simulink library "UAVdesign_net"  (Simulink 7.7)
settings: Solver=ode45  SolverMode=SingleTasking  StartTime=0.0  StopTime=10.0  RelTol=1e-3
undefined symbols (not defined in the file or in its folder): alpha_IERA_IELA_IELA, R_IERA_RA_RA
libraries: UAVdesign_net x75, simulink x13
(part 3 of 8)

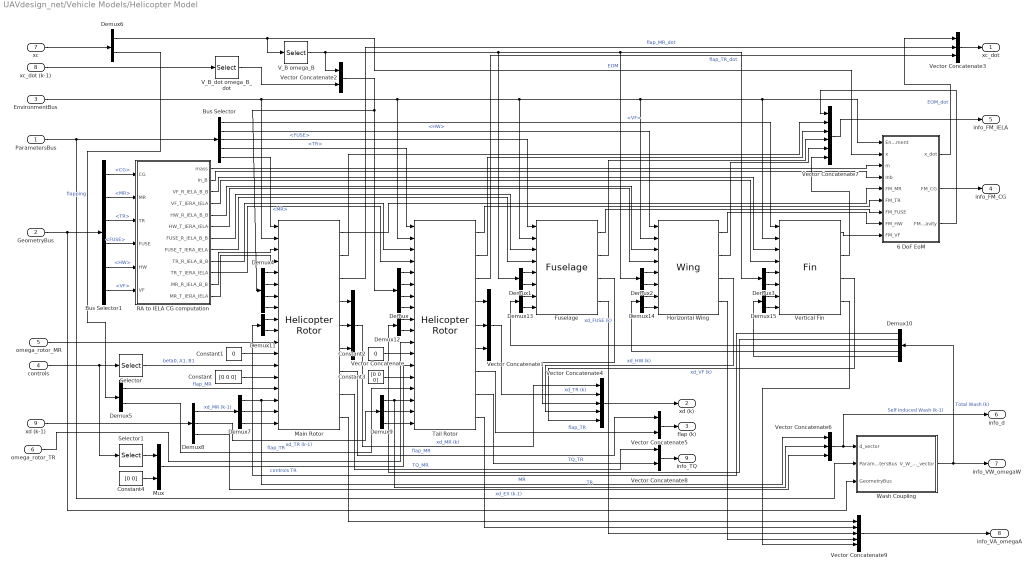
== system UAVdesign_net/Vehicle Models/Helicopter Model ==
  ParametersBus : Inport
  GeometryBus : Inport  Port=2
  EnvironmentBus : Inport  Port=3  OutDataTypeStr=Bus: Environment
  controls : Inport  Port=4
  omega_rotor_MR : Inport  Port=5
  omega_rotor_TR : Inport  Port=6
  xc : Inport  Port=7
  xc_dot (k-1) : Inport  Port=8
  xd (k-1) : Inport  Port=9
  6 DoF EoM : Subsystem
  Bus Selector : BusSelector  OutputSignals=VF,HW,FUSE,TR,MR
  Bus Selector1 : BusSelector  OutputSignals=CG,MR,TR,FUSE,HW,VF
  Constant : Constant  Value=[0 0 0]
  Constant1 : Constant  Value=0
  Constant2 : Constant  Value=0
  Constant3 : Constant  Value=[0 0 0]
  Constant4 : Constant  Value=[0 0]
  Demux : Demux
  Demux{1..3,5,11..15} (9 alike) : Demux  Outputs=2
  Demux10 : Demux  Outputs=[6 6 6 6 6]
  Demux4 : Demux
  Demux6 : Demux  Outputs=[20 6]
  Demux7 : Demux  Outputs=[3 1 1]
  Demux8 : Demux  Outputs=[5 5 9]
  Demux9 : Demux  Outputs=[3 1 1]
  Fuselage : UAVdesign_net/Subsystem Models/Fuselage  SystemSampleTime=-1
  Horizontal Wing : UAVdesign_net/Subsystem Models/Wing  SystemSampleTime=-1
  Main Rotor : UAVdesign_net/Subsystem Models/Helicopter Rotor  SystemSampleTime=-1
  Mux : Mux  Inputs=2
  RA to IELA CG computation : Subsystem
      mask Display:
      | port_label('input', 1, 'CG', 'texmode', 'on')
      | port_label('input', 2, 'MR', 'texmode', 'on')
      | port_label('input', 3, 'TR', 'texmode', 'on')
      | port_label('input', 4, 'FUSE', 'texmode', 'on')
      | port_label('input', 5, 'HW', 'texmode', 'on')
      | port_label('input', 6, 'VF', 'texmode', 'on')
      | 
      | port_label('output', 1, 'mass', 'texmode', 'on')
      | port_label('output', 2, 'In_B', 'texmode', 'on')
      | port_label('output', 3, 'VF R_{IELA-B|B}', 'texmode', 'on')
      | port_label('output', 4, 'VF T_{IERA-IELA}', 'texmode', 'on')
      | port_label('output', 5, 'HW R_{IELA-B|B}', 'texmode', 'on')
      | port_label('output', 6, 'HW T_{IERA-IELA}', 'texmode', 'on')
      | port_label('output', 7, 'FUSE R_{IELA-B|B}', 'texmode', 'on')
      | port_label('output', 8, 'FUSE T_{IERA-IELA}', 'texmode', 'on')
      | port_label('output', 9, 'TR R_{IELA-B|B}', 'texmode', 'on')
      | port_label('output', 10, 'TR T_{IERA-IELA}', 'texmode', 'on')
      | port_label('output', 11, 'MR R_{IELA-B|B}', 'texmode', 'on')
      | port_label('output', 12, 'MR T_{IERA-IELA}', 'texmode', 'on')
  Selector : Selector  InputPortWidth=4  IndexOptions=Index vector (dialog)  Indices=[1:3]  OutputSizes=1
  Selector1 : Selector  InputPortWidth=4  IndexOptions=Index vector (dialog)  Indices=[4]  OutputSizes=1
  Tail Rotor : UAVdesign_net/Subsystem Models/Helicopter Rotor  SystemSampleTime=-1
  V_B omega_B : Selector  InputPortWidth=20  IndexOptions=Index vector (dialog)  Indices=[9:11 15:17]  OutputSizes=1
  V_B_dot omega_B_dot : Selector  InputPortWidth=26  IndexOptions=Index vector (dialog)  Indices=[9:11 15:17]  OutputSizes=1
  Vector Concatenate{,1,3,6} (4 alike) : Concatenate  NumInputs=3  Mode=Vector
  Vector Concatenate2 : Concatenate  Mode=Vector
  Vector Concatenate4 : Concatenate  NumInputs=5  Mode=Vector
  Vector Concatenate5 : Concatenate  Mode=Vector
  Vector Concatenate7 : Concatenate  NumInputs=6  Mode=Vector
  Vector Concatenate8 : Concatenate  Mode=Vector
  Vector Concatenate9 : Concatenate  NumInputs=5  Mode=Vector
  Vertical Fin : UAVdesign_net/Subsystem Models/Fin  SystemSampleTime=-1
  Wash Coupling : Subsystem
      mask Display:
      | port_label('input', 1, 'd VECT', 'texmode', 'on')
      | port_label('input', 2, 'Param.Bus', 'texmode', 'on')
      | port_label('input', 3, 'Geom.Bus', 'texmode', 'on')
      | 
      | port_label('output', 1, 'V_{W} \omega_{W} VECT', 'texmode', 'on')
  xc_dot : Outport
  xd (k) : Outport  Port=2
  flap (k) : Outport  Port=3
  info_FM_CG : Outport  Port=4
  info_FM_IELA : Outport  Port=5
  info_d : Outport  Port=6
  info_VW_omegaW : Outport  Port=7
  info_VA_omegaA : Outport  Port=8
  info_TQ : Outport  Port=9
  wires:
  Vector Concatenate7/1 -> info_FM_IELA/1
  Vertical Fin/2 -> Vector Concatenate7/6
  Horizontal Wing/2 -> Vector Concatenate7/5
  Fuselage/2 -> Vector Concatenate7/4
  Tail Rotor/2 -> Vector Concatenate7/3
  Main Rotor/2 -> Vector Concatenate7/2
  6 DoF EoM/3(FM_Gravity) -> Vector Concatenate7/1
  Fuselage/3 -> Vector Concatenate4/3  "xd_FUSE (k)"
  Tail Rotor/3 -> Vector Concatenate3/3  "flap_TR_dot"
  Tail Rotor/6 -> Vector Concatenate1/3
  Tail Rotor/5 -> Vector Concatenate1/2
  Tail Rotor/4 -> Vector Concatenate1/1
  Tail Rotor/7 -> Vector Concatenate5/2  "flap_TR"
  Main Rotor/3 -> Vector Concatenate3/2  "flap_MR_dot"
  Main Rotor/6 -> Vector Concatenate/3
  Main Rotor/5 -> Vector Concatenate/2
  Main Rotor/4 -> Vector Concatenate/1
  Main Rotor/7 -> Vector Concatenate5/1  "flap_MR"
  Horizontal Wing/3 -> Vector Concatenate4/4  "xd_HW (k)"
  Vertical Fin/3 -> Vector Concatenate4/5  "xd_VF (k)"
  Demux10/1 -> Demux11/1
  Demux10/2 -> Demux12/1
  Demux10/3 -> Demux13/1
  Demux10/4 -> Demux14/1
  Demux10/5 -> Demux15/1
  Vector Concatenate6/1 -> info_d/1, Wash Coupling/1(d_vector)  "Self Induced Wash (k-1)"
  Wash Coupling/1(V_W_omega_W_vector) -> Demux10/1, info_VW_omegaW/1  "Total Wash (k)"
  Demux15/2 -> Vertical Fin/8
  Demux15/1 -> Vertical Fin/7
  Demux14/2 -> Horizontal Wing/8
  Demux14/1 -> Horizontal Wing/7
  Demux13/2 -> Fuselage/8
  Demux13/1 -> Fuselage/7
  Demux12/2 -> Tail Rotor/10
  Demux12/1 -> Tail Rotor/9
  Demux11/2 -> Main Rotor/10
  Demux11/1 -> Main Rotor/9
  6 DoF EoM/2(FM_CG) -> info_FM_CG/1
  Vector Concatenate5/1 -> flap (k)/1
  Demux1/1 -> Fuselage/5
  Demux1/2 -> Fuselage/6
  Demux3/2 -> Vertical Fin/6
  Demux3/1 -> Vertical Fin/5
  Demux2/2 -> Horizontal Wing/6
  Demux2/1 -> Horizontal Wing/5
  Demux8/3 -> Vector Concatenate6/3  "xd_EX (k-1)"
  xd (k-1)/1 -> Demux8/1
  Vector Concatenate/1 -> Vector Concatenate4/1  "xd_MR (k)"
  Demux8/2 -> Demux9/1  "xd_TR (k-1)"
  Demux8/1 -> Demux7/1  "xd_MR (k-1)"
  Demux5/1 -> Main Rotor/15  "flap_MR"
  Demux9/3 -> Tail Rotor/18
  Demux9/2 -> Tail Rotor/17
  Vector Concatenate4/1 -> xd (k)/1
  Vector Concatenate1/1 -> Vector Concatenate4/2  "xd_TR (k)"
  Demux7/3 -> Main Rotor/18
  Demux7/2 -> Main Rotor/17
  Demux5/2 -> Tail Rotor/15  "flap_TR"
  6 DoF EoM/1(x_dot) -> Vector Concatenate3/1  "EOM_dot"
  Vector Concatenate3/1 -> xc_dot/1
  Vector Concatenate2/1 -> Demux4/1, Demux/1
  V_B_dot omega_B_dot/1 -> Vector Concatenate2/2
  V_B omega_B/1 -> Demux2/1, Demux3/1, Demux1/1, Vector Concatenate2/1
  Demux6/1 -> V_B omega_B/1, 6 DoF EoM/2(x)  "EOM"
  Demux6/2 -> Demux5/1  "flapping"
  xc/1 -> Demux6/1
  xc_dot (k-1)/1 -> V_B_dot omega_B_dot/1
  GeometryBus/1 -> Wash Coupling/3(GeometryBus), Bus Selector1/1
  Bus Selector1/6 -> RA to IELA CG computation/6(VF)  "<VF>"
  Bus Selector1/5 -> RA to IELA CG computation/5(HW)  "<HW>"
  Bus Selector1/4 -> RA to IELA CG computation/4(FUSE)  "<FUSE>"
  Bus Selector1/3 -> RA to IELA CG computation/3(TR)  "<TR>"
  Bus Selector1/2 -> RA to IELA CG computation/2(MR)  "<MR>"
  Bus Selector1/1 -> RA to IELA CG computation/1(CG)  "<CG>"
  EnvironmentBus/1 -> Main Rotor/2, Tail Rotor/2, Fuselage/2, Horizontal Wing/2, Vertical Fin/2, 6 DoF EoM/1(Environment)
  ParametersBus/1 -> Wash Coupling/2(ParametersBus), Bus Selector/1
  Bus Selector/1 -> Vertical Fin/1  "<VF>"
  Bus Selector/2 -> Horizontal Wing/1  "<HW>"
  Bus Selector/3 -> Fuselage/1  "<FUSE>"
  Bus Selector/4 -> Tail Rotor/1  "<TR>"
  Bus Selector/5 -> Main Rotor/1  "<MR>"
  Constant4/1 -> Mux/2
  Selector1/1 -> Mux/1
  Mux/1 -> Tail Rotor/13  "controls TR"
  omega_rotor_TR/1 -> Tail Rotor/11
  Constant3/1 -> Tail Rotor/14
  Constant2/1 -> Tail Rotor/12
  controls/1 -> Selector/1, Selector1/1
  Selector/1 -> Main Rotor/13  "beta0, A1, B1"
  omega_rotor_MR/1 -> Main Rotor/11
  Constant1/1 -> Main Rotor/12
  Constant/1 -> Main Rotor/14
  Demux4/4 -> Main Rotor/8
  Demux4/3 -> Main Rotor/7
  Demux4/2 -> Main Rotor/6
  Demux4/1 -> Main Rotor/5
  Demux/4 -> Tail Rotor/8
  Demux/3 -> Tail Rotor/7
  Demux/2 -> Tail Rotor/6
  Demux/1 -> Tail Rotor/5
  RA to IELA CG computation/10(TR_T_IERA_IELA) -> Tail Rotor/4
  RA to IELA CG computation/9(TR_R_IELA_B_B) -> Tail Rotor/3
  RA to IELA CG computation/8(FUSE_T_IERA_IELA) -> Fuselage/4
  RA to IELA CG computation/7(FUSE_R_IELA_B_B) -> Fuselage/3
  RA to IELA CG computation/6(HW_T_IERA_IELA) -> Horizontal Wing/4
  RA to IELA CG computation/5(HW_R_IELA_B_B) -> Horizontal Wing/3
  RA to IELA CG computation/4(VF_T_IERA_IELA) -> Vertical Fin/4
  RA to IELA CG computation/3(VF_R_IELA_B_B) -> Vertical Fin/3
  Tail Rotor/1 -> 6 DoF EoM/6(FM_TR)
  Fuselage/1 -> 6 DoF EoM/7(FM_FUSE)
  Horizontal Wing/1 -> 6 DoF EoM/8(FM_HW)
  Vertical Fin/1 -> 6 DoF EoM/9(FM_VF)
  Demux9/1 -> Vector Concatenate6/2, Tail Rotor/16  "TR"
  Demux7/1 -> Vector Concatenate6/1, Main Rotor/16  "MR"
  RA to IELA CG computation/2(In_B) -> 6 DoF EoM/4(Inb)
  RA to IELA CG computation/1(mass) -> 6 DoF EoM/3(m)
  Main Rotor/1 -> 6 DoF EoM/5(FM_MR)
  RA to IELA CG computation/11(MR_R_IELA_B_B) -> Main Rotor/3
  RA to IELA CG computation/12(MR_T_IERA_IELA) -> Main Rotor/4
  Tail Rotor/8 -> Vector Concatenate8/2  "TQ_TR"
  Main Rotor/8 -> Vector Concatenate8/1  "TQ_MR"
  Vector Concatenate8/1 -> info_TQ/1
  Main Rotor/9 -> Vector Concatenate9/1
  Tail Rotor/9 -> Vector Concatenate9/2
  Fuselage/4 -> Vector Concatenate9/3
  Horizontal Wing/4 -> Vector Concatenate9/4
  Vertical Fin/4 -> Vector Concatenate9/5
  Vector Concatenate9/1 -> info_VA_omegaA/1

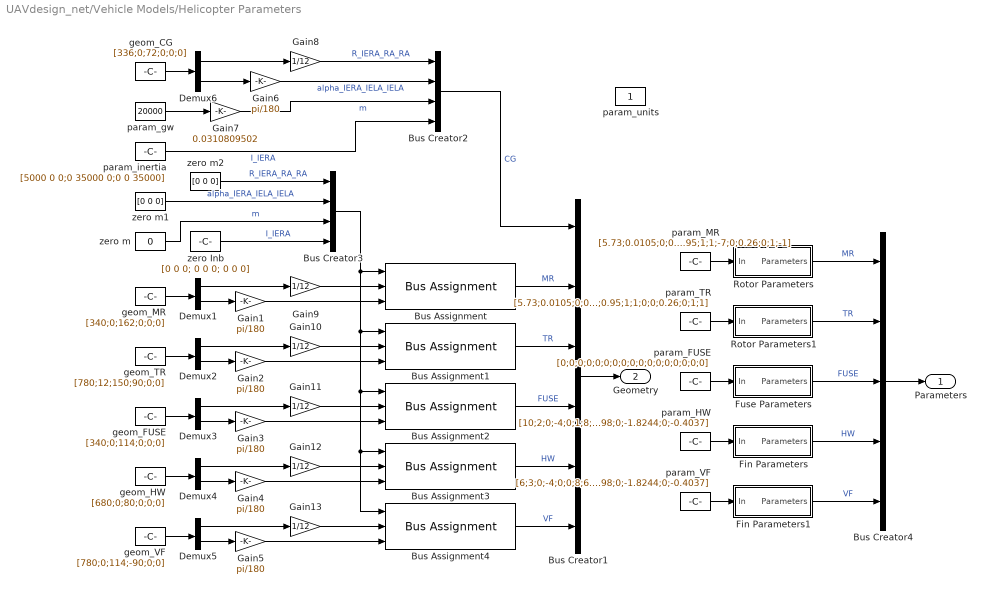
== system UAVdesign_net/Vehicle Models/Helicopter Parameters ==
  Bus Assignment{,1..4} (5 alike) : BusAssignment  AssignedSignals=R_IERA_RA_RA,alpha_IERA_IELA_IELA
  Bus Creator1 : BusCreator  Inputs=6
  Bus Creator2 : BusCreator  OutDataTypeStr=Bus: GeometryParameters
  Bus Creator3 : BusCreator  OutDataTypeStr=Bus: GeometryParameters
  Bus Creator4 : BusCreator  Inputs=5
  Demux{1..6} (6 alike) : Demux  Outputs=2
  Fin Parameters : Subsystem
  Fin Parameters1 : Subsystem
  Fuse Parameters : Subsystem
  Gain{1..6} (6 alike) : Gain  Gain=pi/180
  Gain{8..13} (6 alike) : Gain  Gain=1/12
  Gain7 : Gain  Gain=0.0310809502
  Rotor Parameters : Subsystem
  Rotor Parameters1 : Subsystem
  geom_CG : Constant  Value=[336;0;72;0;0;0]
  geom_FUSE : Constant  Value=[340;0;114;0;0;0]
  geom_HW : Constant  Value=[680;0;80;0;0;0]
  geom_MR : Constant  Value=[340;0;162;0;0;0]
  geom_TR : Constant  Value=[780;12;150;90;0;0]
  geom_VF : Constant  Value=[780;0;114;-90;0;0]
  param_FUSE : Constant  Value=[0;0;0;0;0;0;0;0;0;0;0;0;0;0;0;0;0]
  param_HW : Constant  Value=[10;2;0;-4;0;1;8;6.13;0.9682;1.8898;0;-1.8244;0;-0.4037]
  param_MR : Constant  Value=[5.73;0.0105;0;0.01325;0;-15;0;0;7;30;2.5;0.95;1;1;-7;0;0.26;0;1;-1]
  param_TR : Constant  Value=[5.73;0.0105;0;0.01325;0;-45;0;0;4;6.5;1.25;0.95;1;1;0;0;0.26;0;1;1]
  param_VF : Constant  Value=[6;3;0;-4;0;0;8;6.1311;0.9682;1.8898;0;-1.8244;0;-0.4037]
  param_gw : Constant  Value=20000
  param_inertia : Constant  Value=[5000 0 0;0 35000 0;0 0 35000]
  param_units : Constant
  zero Inb : Constant  Value=[0 0 0; 0 0 0; 0 0 0]
  zero m : Constant  Value=0
  zero m1 : Constant  Value=[0 0 0]
  zero m2 : Constant  Value=[0 0 0]
  Parameters : Outport
  Geometry : Outport  Port=2
  wires:
  Bus Creator2/1 -> Bus Creator1/1  "CG"
  Bus Assignment1/1 -> Bus Creator1/3  "TR"
  Bus Assignment2/1 -> Bus Creator1/4  "FUSE"
  Bus Assignment3/1 -> Bus Creator1/5  "HW"
  Bus Assignment4/1 -> Bus Creator1/6  "VF"
  Bus Creator1/1 -> Geometry/1
  Demux6/1 -> Gain8/1
  Demux6/2 -> Gain6/1
  param_gw/1 -> Gain7/1
  param_inertia/1 -> Bus Creator2/4  "I_IERA"
  Bus Assignment/1 -> Bus Creator1/2  "MR"
  Demux1/1 -> Gain9/1
  Demux1/2 -> Gain1/1
  geom_MR/1 -> Demux1/1
  Demux2/1 -> Gain10/1
  Demux2/2 -> Gain2/1
  geom_TR/1 -> Demux2/1
  Demux3/1 -> Gain11/1
  Demux3/2 -> Gain3/1
  geom_FUSE/1 -> Demux3/1
  Demux4/1 -> Gain12/1
  Demux4/2 -> Gain4/1
  geom_HW/1 -> Demux4/1
  Demux5/1 -> Gain13/1
  Demux5/2 -> Gain5/1
  geom_VF/1 -> Demux5/1
  geom_CG/1 -> Demux6/1
  Bus Creator3/1 -> Bus Assignment/1, Bus Assignment1/1, Bus Assignment2/1, Bus Assignment4/1, Bus Assignment3/1
  zero m/1 -> Bus Creator3/3  "m"
  zero m1/1 -> Bus Creator3/2  "alpha_IERA_IELA_IELA"
  zero Inb/1 -> Bus Creator3/4  "I_IERA"
  zero m2/1 -> Bus Creator3/1  "R_IERA_RA_RA"
  Bus Creator4/1 -> Parameters/1
  Rotor Parameters/1(Parameters) -> Bus Creator4/1  "MR"
  param_MR/1 -> Rotor Parameters/1(In)
  Rotor Parameters1/1(Parameters) -> Bus Creator4/2  "TR"
  param_TR/1 -> Rotor Parameters1/1(In)
  param_FUSE/1 -> Fuse Parameters/1(In)
  Fuse Parameters/1(Parameters) -> Bus Creator4/3  "FUSE"
  param_VF/1 -> Fin Parameters1/1(In)
  Fin Parameters1/1(Parameters) -> Bus Creator4/5  "VF"
  Fin Parameters/1(Parameters) -> Bus Creator4/4  "HW"
  param_HW/1 -> Fin Parameters/1(In)
  Gain1/1 -> Bus Assignment/3
  Gain2/1 -> Bus Assignment1/3
  Gain3/1 -> Bus Assignment2/3
  Gain4/1 -> Bus Assignment3/3
  Gain5/1 -> Bus Assignment4/3
  Gain6/1 -> Bus Creator2/2  "alpha_IERA_IELA_IELA"
  Gain7/1 -> Bus Creator2/3  "m"
  Gain8/1 -> Bus Creator2/1  "R_IERA_RA_RA"
  Gain9/1 -> Bus Assignment/2
  Gain10/1 -> Bus Assignment1/2
  Gain11/1 -> Bus Assignment2/2
  Gain12/1 -> Bus Assignment3/2
  Gain13/1 -> Bus Assignment4/2

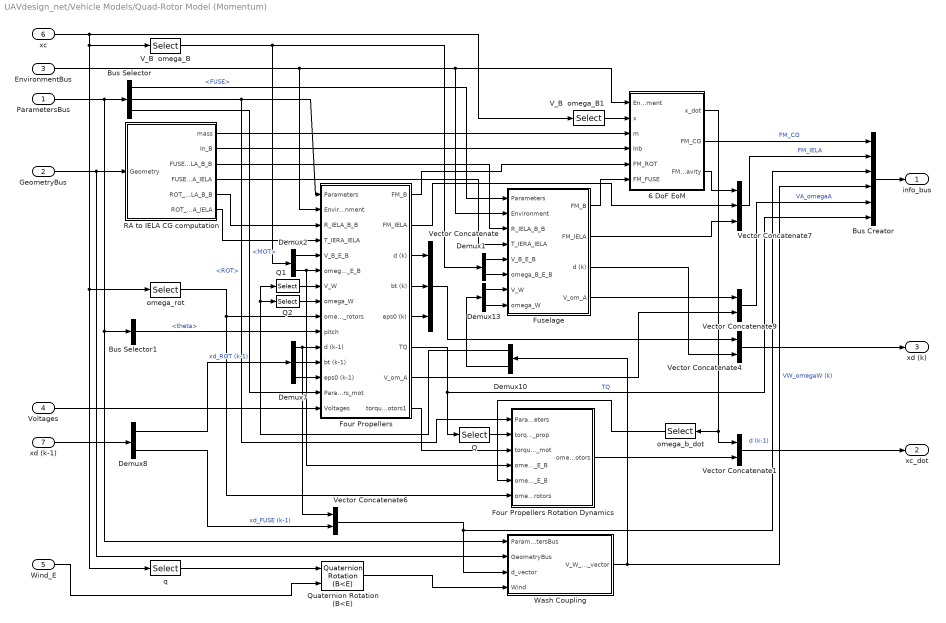
== system UAVdesign_net/Vehicle Models/Quad-Rotor Model (Momentum) ==
  ParametersBus : Inport
  GeometryBus : Inport  Port=2
  EnvironmentBus : Inport  Port=3
  Voltages : Inport  Port=4
  Wind_E : Inport  Port=5
  xc : Inport  Port=6
  xd (k-1) : Inport  Port=7
  6 DoF EoM : Subsystem
  Bus Creator : BusCreator  Inputs=6
  Bus Selector : BusSelector  OutputSignals=FUSE,ROT,MOT
  Bus Selector1 : BusSelector  OutputSignals=ROT.theta
  Demux1 : Demux  Outputs=2
  Demux10 : Demux  Outputs=[24 6]
  Demux13 : Demux  Outputs=2
  Demux2 : Demux  Outputs=2
  Demux7 : Demux  Outputs=[12 4 4]
  Demux8 : Demux  Outputs=[20 3]
  Four Propellers : Subsystem  TreatAsAtomicUnit=on
      mask Display:
      | port_label('input', 1, 'Parameters', 'texmode', 'on')
      | port_label('input', 2, 'Environment', 'texmode', 'on')
      | port_label('input', 3, 'R_{IELA-B|B}', 'texmode', 'on')
      | port_label('input', 4, 'T_{IERA-IELA}', 'texmode', 'on')
      | port_label('input', 5, 'V_{B-E|B}', 'texmode', 'on')
      | port_label('input', 6, '\omega_{B-E|B}', 'texmode', 'on')
      | port_label('input', 7, 'V_{W|B}', 'texmode', 'on')
      | port_label('input', 8, '\omega_{W|B}', 'texmode', 'on')
      | port_label('input', 9, '\Omega_{rotor}', 'texmode', 'on')
      | port_label('input', 10, 'pitch', 'texmode', 'on')
      | port_label('input', 11, 'd_{k-1|IELA}', 'texmode', 'on')
      | port_label('input', 12, 'bt_{k-1}', 'texmode', 'on')
      | port_label('input', 13, 'eps0_{k-1}', 'texmode', 'on')
      | port_label('input', 14, 'Parameters_{mot}', 'texmode', 'on')
      | port_label('input', 15, 'V_{mot}', 'texmode', 'on')
      | 
      | port_label('output', 1, 'FM_{B}', 'texmode', 'on')
      | port_label('output', 2, 'FM_{IELA}', 'texmode', 'on')
      | port_label('output', 3, 'd_{k|IELA}', 'texmode', 'on')
      | port_label('output', 4, 'bt_{k}', 'texmode', 'on')
      | port_label('output', 5, 'eps0_{k}', 'texmode', 'on')
      | port_label('output', 6, 'T Q', 'texmode', 'on')
      | port_label('output', 7, 'V \omega_{A|IELA}', 'texmode', 'on')
      | port_label('output', 8, '\tau_{motor}', 'texmode', 'on')
  Four Propellers Rotation Dynamics : Subsystem  TreatAsAtomicUnit=on
      mask Display:
      | port_label('input', 1, 'Parameters', 'texmode', 'on')
      | port_label('input', 2, '\tau_{prop} (Q)', 'texmode', 'on')
      | port_label('input', 3, '\tau_{motor}', 'texmode', 'on')
      | port_label('input', 4, '\omega_{B-E|B}', 'texmode', 'on')
      | port_label('input', 5, '\omega^\bullet_{B-E|B}', 'texmode', 'on')
      | port_label('input', 6, '\Omega_{rotor}', 'texmode', 'on')
      | 
      | port_label('output', 1, '\Omega^\bullet_{rotor}', 'texmode', 'on')
  Fuselage : Subsystem  TreatAsAtomicUnit=on
      mask Type: HelicopterFuselageModel
      mask Description: Fuselage model.
      mask Display:
      | port_label('input', 1, 'Parameters', 'texmode', 'on')
      | port_label('input', 2, 'Environment', 'texmode', 'on')
      | port_label('input', 3, 'R_{IELA-B|B}', 'texmode', 'on')
      | port_label('input', 4, 'T_{IERA-IELA}', 'texmode', 'on')
      | port_label('input', 5, 'V_{B-E|B}', 'texmode', 'on')
      | port_label('input', 6, '\omega_{B-E|B}', 'texmode', 'on')
      | port_label('input', 7, 'V_{W|B}', 'texmode', 'on')
      | port_label('input', 8, '\omega_{W|B}', 'texmode', 'on')
      | 
      | port_label('output', 1, 'FM_{B}', 'texmode', 'on')
      | port_label('output', 2, 'FM_{IELA}', 'texmode', 'on')
      | port_label('output', 3, 'd_{IELA}', 'texmode', 'on')
      | port_label('output', 4, 'V \omega_{A|IELA}', 'texmode', 'on')
  Q : Selector  InputPortWidth=8  IndexOptions=Index vector (dialog)  Indices=[2 4 6 8]  OutputSizes=1
  Q1 : Selector  InputPortWidth=24  IndexOptions=Index vector (dialog)  Indices=[1:3 7:9 13:15 19:21]  OutputSizes=1
  Q2 : Selector  InputPortWidth=24  IndexOptions=Index vector (dialog)  Indices=[4:6 10:12 16:18 22:24]  OutputSizes=1
  Quaternion Rotation (B<E) : UAVdesign_net/Utilities/Math/Quaternion Rotation (B<E)  SystemSampleTime=-1
  RA to IELA CG computation : Subsystem
      mask Display:
      | port_label('input', 1, 'Geom', 'texmode', 'on')
      | 
      | port_label('output', 1, 'mass', 'texmode', 'on')
      | port_label('output', 2, 'In_B', 'texmode', 'on')
      | port_label('output', 3, 'FUSE R_{IELA-B|B}', 'texmode', 'on')
      | port_label('output', 4, 'FUSE T_{IERA-IELA}', 'texmode', 'on')
      | port_label('output', 5, 'ROT R_{IELA-B|B}', 'texmode', 'on')
      | port_label('output', 6, 'ROT T_{IERA-IELA}', 'texmode', 'on')
  V_B  omega_B : Selector  InputPortWidth=17  IndexOptions=Index vector (dialog)  Indices=[1:6]  OutputSizes=1
  V_B  omega_B1 : Selector  InputPortWidth=17  IndexOptions=Index vector (dialog)  Indices=[1:13]  OutputSizes=1
  Vector Concatenate : Concatenate  NumInputs=3  Mode=Vector
  Vector Concatenate{1,4,6,9} (4 alike) : Concatenate  Mode=Vector
  Vector Concatenate7 : Concatenate  NumInputs=3  Mode=Vector
  Wash Coupling : Subsystem
      mask Display:
      | port_label('input', 1, 'Param.Bus', 'texmode', 'on')
      | port_label('input', 2, 'Geom.Bus', 'texmode', 'on')
      | port_label('input', 3, 'd VECT', 'texmode', 'on')
      | port_label('input', 4, 'wind VECT', 'texmode', 'on')
      | 
      | port_label('output', 1, 'V_{W} \omega_{W} VECT', 'texmode', 'on')
  omega_b_dot : Selector  InputPortWidth=13  IndexOptions=Index vector (dialog)  Indices=[4:6]  OutputSizes=1
  omega_rot : Selector  InputPortWidth=17  IndexOptions=Index vector (dialog)  Indices=[14:17]  OutputSizes=1
  q : Selector  InputPortWidth=17  IndexOptions=Index vector (dialog)  Indices=[10:13]  OutputSizes=1
  info_bus : Outport
  xc_dot : Outport  Port=2
  xd (k) : Outport  Port=3
  wires:
  Vector Concatenate9/1 -> Bus Creator/5  "VA_omegaA"
  Four Propellers/1(FM_B) -> 6 DoF EoM/5(FM_ROT)
  RA to IELA CG computation/1(mass) -> 6 DoF EoM/3(m)
  RA to IELA CG computation/2(In_B) -> 6 DoF EoM/4(Inb)
  Fuselage/1(FM_B) -> 6 DoF EoM/6(FM_FUSE)
  RA to IELA CG computation/3(FUSE_R_IELA_B_B) -> Fuselage/3(R_IELA_B_B)
  RA to IELA CG computation/4(FUSE_T_IERA_IELA) -> Fuselage/4(T_IERA_IELA)
  Bus Selector/2 -> Four Propellers/1(Parameters), Four Propellers Rotation Dynamics/1(Parameters)  "<ROT>"
  Bus Selector/1 -> Fuselage/1(Parameters)  "<FUSE>"
  ParametersBus/1 -> Bus Selector/1, Wash Coupling/1(ParametersBus), Bus Selector1/1
  EnvironmentBus/1 -> Fuselage/2(Environment), 6 DoF EoM/1(Environment), Four Propellers/2(Environment)
  GeometryBus/1 -> Wash Coupling/2(GeometryBus), RA to IELA CG computation/1(Geometry)
  V_B  omega_B/1 -> Demux1/1, Demux2/1
  Vector Concatenate4/1 -> xd (k)/1
  Demux8/1 -> Demux7/1  "xd_ROT (k-1)"
  xd (k-1)/1 -> Demux8/1
  Demux1/2 -> Fuselage/6(omega_B_E_B)
  Demux1/1 -> Fuselage/5(V_B_E_B)
  Demux13/1 -> Fuselage/7(V_W)
  Demux13/2 -> Fuselage/8(omega_W)
  Wash Coupling/1(V_W_omega_W_vector) -> Demux10/1, Bus Creator/4  "VW_omegaW (k)"
  Demux10/1 -> Q1/1, Q2/1
  6 DoF EoM/3(FM_Gravity) -> Vector Concatenate7/1
  Four Propellers/2(FM_IELA) -> Vector Concatenate7/2
  Fuselage/2(FM_IELA) -> Vector Concatenate7/3
  Vector Concatenate7/1 -> Bus Creator/2  "FM_IELA"
  Four Propellers/3(d (k)) -> Vector Concatenate/1
  Fuselage/4(V_om_A) -> Vector Concatenate9/1
  Demux10/2 -> Demux13/1
  Vector Concatenate/1 -> Vector Concatenate4/1
  Fuselage/3(d (k)) -> Vector Concatenate4/2
  Demux8/2 -> Vector Concatenate6/2  "xd_FUSE (k-1)"
  Vector Concatenate6/1 -> Wash Coupling/3(d_vector), Bus Creator/3  "d (k-1)"
  xc/1 -> V_B  omega_B/1, omega_rot/1, q/1, V_B  omega_B1/1
  RA to IELA CG computation/5(ROT_R_IELA_B_B) -> Four Propellers/3(R_IELA_B_B)
  Bus Selector1/1 -> Four Propellers/10(pitch)  "<theta>"
  RA to IELA CG computation/6(ROT_T_IERA_IELA) -> Four Propellers/4(T_IERA_IELA)
  Demux2/1 -> Four Propellers/5(V_B_E_B)
  Demux2/2 -> Four Propellers/6(omega_B_E_B), Four Propellers Rotation Dynamics/4(omega_B_E_B)
  Q1/1 -> Four Propellers/7(V_W)
  Q2/1 -> Four Propellers/8(omega_W)
  Demux7/1 -> Four Propellers/11(d (k-1)), Vector Concatenate6/1
  Demux7/2 -> Four Propellers/12(bt (k-1))
  Demux7/3 -> Four Propellers/13(eps0 (k-1))
  Bus Selector/3 -> Four Propellers/14(Parameters_mot)  "<MOT>"
  Voltages/1 -> Four Propellers/15(Voltages)
  Four Propellers/7(V_om_A) -> Vector Concatenate9/2
  Four Propellers/4(bt (k)) -> Vector Concatenate/2
  Four Propellers/5(eps0 (k)) -> Vector Concatenate/3
  Four Propellers/8(torque_motors1) -> Four Propellers Rotation Dynamics/3(torque_mot)
  Q/1 -> Four Propellers Rotation Dynamics/2(torque_prop)
  Four Propellers/6(TQ) -> Q/1, Bus Creator/6  "TQ"
  6 DoF EoM/1(x_dot) -> Vector Concatenate1/1, omega_b_dot/1
  Vector Concatenate1/1 -> xc_dot/1
  Four Propellers Rotation Dynamics/1(omega_dot_motors) -> Vector Concatenate1/2
  omega_b_dot/1 -> Four Propellers Rotation Dynamics/5(omega_dot_B_E_B)
  omega_rot/1 -> Four Propellers/9(omega_rotors), Four Propellers Rotation Dynamics/6(omega_rotors)
  Bus Creator/1 -> info_bus/1
  6 DoF EoM/2(FM_CG) -> Bus Creator/1  "FM_CG"
  V_B  omega_B1/1 -> 6 DoF EoM/2(x)
  Quaternion Rotation (B<E)/1 -> Wash Coupling/4(Wind)
  Wind_E/1 -> Quaternion Rotation (B<E)/2
  q/1 -> Quaternion Rotation (B<E)/1

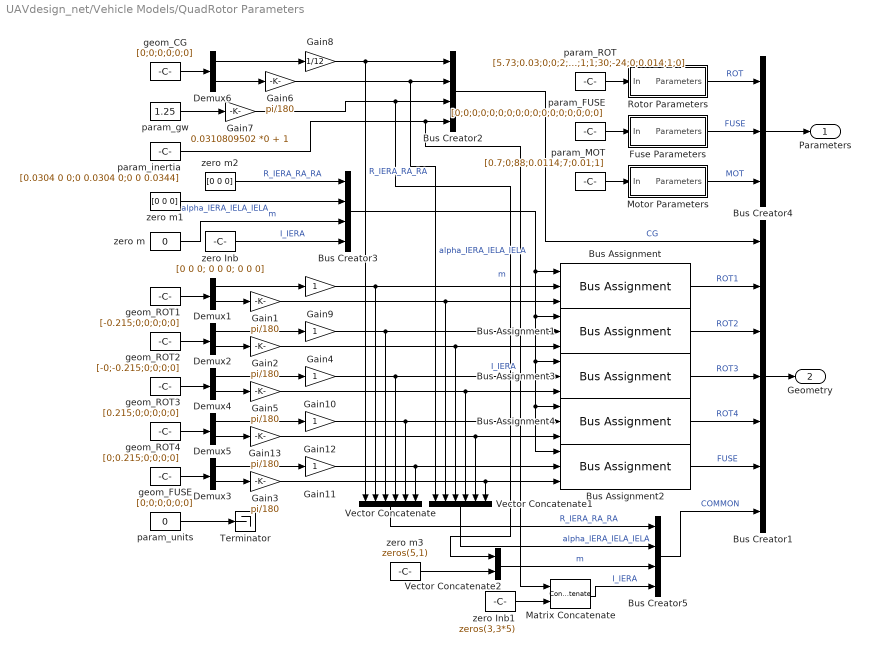
== system UAVdesign_net/Vehicle Models/QuadRotor Parameters ==
  Bus Assignment{,1..4} (5 alike) : BusAssignment  AssignedSignals=R_IERA_RA_RA,alpha_IERA_IELA_IELA
  Bus Creator1 : BusCreator  Inputs=7
  Bus Creator2 : BusCreator
  Bus Creator3 : BusCreator
  Bus Creator4 : BusCreator  Inputs=3
  Bus Creator5 : BusCreator
  Demux{1..6} (6 alike) : Demux  Outputs=2
  Fuse Parameters : Subsystem
  Gain{1..3,5..6,13} (6 alike) : Gain  Gain=pi/180
  Gain{4,9..12} (5 alike) : Gain
  Gain7 : Gain  Gain=0.0310809502 *0 + 1
  Gain8 : Gain  Gain=1/12
  Matrix Concatenate : Concatenate  Mode=Multidimensional array  ConcatenateDimension=2
  Motor Parameters : Subsystem
  Rotor Parameters : Subsystem
  Terminator : Terminator
  Vector Concatenate : Concatenate  NumInputs=6  Mode=Vector
  Vector Concatenate1 : Concatenate  NumInputs=6  Mode=Vector
  Vector Concatenate2 : Concatenate  Mode=Vector
  geom_CG : Constant  Value=[0;0;0;0;0;0]
  geom_FUSE : Constant  Value=[0;0;0;0;0;0]
  geom_ROT1 : Constant  Value=[-0.215;0;0;0;0;0]
  geom_ROT2 : Constant  Value=[-0;-0.215;0;0;0;0]
  geom_ROT3 : Constant  Value=[0.215;0;0;0;0;0]
  geom_ROT4 : Constant  Value=[0;0.215;0;0;0;0]
  param_FUSE : Constant  Value=[0;0;0;0;0;0;0;0;0;0;0;0;0;0;0;0;0]
  param_MOT : Constant  Value=[0.7;0;88;0.0114;7;0.01;1]
  param_ROT : Constant  Value=[5.73;0.03;0;0;2;0.127;0.016;0.95;1;1;30;-24;0;0.014;1;0]
  param_gw : Constant  Value=1.25
  param_inertia : Constant  Value=[0.0304 0 0;0 0.0304 0;0 0 0.0344]
  param_units : Constant  Value=0
  zero Inb : Constant  Value=[0 0 0; 0 0 0; 0 0 0]
  zero Inb1 : Constant  Value=zeros(3,3*5)
  zero m : Constant  Value=0
  zero m1 : Constant  Value=[0 0 0]
  zero m2 : Constant  Value=[0 0 0]
  zero m3 : Constant  Value=zeros(5,1)
  Parameters : Outport
  Geometry : Outport  Port=2
  wires:
  Motor Parameters/1(Parameters) -> Bus Creator4/3  "MOT"
  param_MOT/1 -> Motor Parameters/1(In)
  zero Inb1/1 -> Matrix Concatenate/2
  Vector Concatenate/1 -> Bus Creator5/1  "R_IERA_RA_RA"
  Matrix Concatenate/1 -> Bus Creator5/4  "I_IERA"
  Vector Concatenate1/1 -> Bus Creator5/2  "alpha_IERA_IELA_IELA"
  Bus Creator5/1 -> Bus Creator1/7  "COMMON"
  Bus Assignment4/1 -> Bus Creator1/5  "ROT4"
  Bus Assignment3/1 -> Bus Creator1/4  "ROT3"
  Bus Assignment1/1 -> Bus Creator1/3  "ROT2"
  geom_ROT4/1 -> Demux5/1
  Gain12/1 -> Vector Concatenate/5, Bus Assignment4/2
  Gain13/1 -> Vector Concatenate1/5, Bus Assignment4/3
  Demux5/2 -> Gain13/1
  Demux5/1 -> Gain12/1
  geom_ROT3/1 -> Demux4/1
  Gain10/1 -> Vector Concatenate/4, Bus Assignment3/2
  Gain5/1 -> Vector Concatenate1/4, Bus Assignment3/3
  Demux4/2 -> Gain5/1
  Demux4/1 -> Gain10/1
  Gain9/1 -> Vector Concatenate/2, Bus Assignment/2
  geom_ROT2/1 -> Demux2/1
  Gain4/1 -> Vector Concatenate/3, Bus Assignment1/2
  Gain2/1 -> Vector Concatenate1/3, Bus Assignment1/3
  Demux2/2 -> Gain2/1
  Demux2/1 -> Gain4/1
  param_inertia/1 -> Matrix Concatenate/1, Bus Creator2/4  "I_IERA"
  Gain7/1 -> Bus Creator2/3, Vector Concatenate2/1  "m"
  zero m/1 -> Bus Creator3/3  "m"
  zero Inb/1 -> Bus Creator3/4  "I_IERA"
  Gain6/1 -> Vector Concatenate1/1, Bus Creator2/2  "alpha_IERA_IELA_IELA"
  Gain8/1 -> Vector Concatenate/1, Bus Creator2/1  "R_IERA_RA_RA"
  Fuse Parameters/1(Parameters) -> Bus Creator4/2  "FUSE"
  Rotor Parameters/1(Parameters) -> Bus Creator4/1  "ROT"
  param_units/1 -> Terminator/1
  zero m1/1 -> Bus Creator3/2  "alpha_IERA_IELA_IELA"
  zero m2/1 -> Bus Creator3/1  "R_IERA_RA_RA"
  Bus Creator2/1 -> Bus Creator1/1  "CG"
  Bus Assignment/1 -> Bus Creator1/2  "ROT1"
  Bus Assignment2/1 -> Bus Creator1/6  "FUSE"
  Gain11/1 -> Vector Concatenate/6, Bus Assignment2/2
  Gain3/1 -> Vector Concatenate1/6, Bus Assignment2/3
  Gain1/1 -> Vector Concatenate1/2, Bus Assignment/3
  param_FUSE/1 -> Fuse Parameters/1(In)
  param_ROT/1 -> Rotor Parameters/1(In)
  Bus Creator4/1 -> Parameters/1
  Bus Creator3/1 -> Bus Assignment4/1, Bus Assignment2/1, Bus Assignment3/1, Bus Assignment1/1, Bus Assignment/1
  geom_CG/1 -> Demux6/1
  geom_FUSE/1 -> Demux3/1
  Demux3/2 -> Gain3/1
  Demux3/1 -> Gain11/1
  geom_ROT1/1 -> Demux1/1
  Demux1/2 -> Gain1/1
  Demux1/1 -> Gain9/1
  param_gw/1 -> Gain7/1
  Demux6/2 -> Gain6/1
  Demux6/1 -> Gain8/1
  Bus Creator1/1 -> Geometry/1
  Vector Concatenate2/1 -> Bus Creator5/3  "m"
  zero m3/1 -> Vector Concatenate2/2

== system UAVdesign_net/Subsystem Models/Fin/CG to IELA ==
  R_IELA-B|B : Inport
  V_B-E|B : Inport  Port=2
  omega_B_E|B : Inport  Port=3
  3x3 Cross Product : UAVdesign_net/Utilities/Math/3x3 Cross Product  SystemSampleTime=-1
  Sum : Sum  Inputs=++|
  V_IELA-E|IELA : Outport
  omega_IELA-E|IELA : Outport  Port=2
  wires:
  omega_B_E|B/1 -> 3x3 Cross Product/1, omega_IELA-E|IELA/1
  R_IELA-B|B/1 -> 3x3 Cross Product/2
  3x3 Cross Product/1 -> Sum/2
  V_B-E|B/1 -> Sum/1
  Sum/1 -> V_IELA-E|IELA/1

== system UAVdesign_net/Subsystem Models/Fin/Fin Model (IERA) ==
  Parameters : Inport  OutDataTypeStr=Bus: FinParameters
  Environment : Inport  Port=2  OutDataTypeStr=Bus: Environment
  V_A : Inport  Port=3
  omega_A : Inport  Port=4
  V_W : Inport  Port=5
  omega_W : Inport  Port=6
  control : Inport  Port=7
  Bus Selector : BusSelector  OutputSignals=dihedral,incid,sweep
  Euler Rotation Matrix MAC to WRA (Half Wing) : UAVdesign_net/Utilities/Axes/Euler Rotation Matrix from Earth to Body  SystemSampleTime=-1
  Fin : Subsystem
      mask Display:
      | port_label('input', 1, 'Parameters', 'texmode', 'on')
      | port_label('input', 2, 'Environment', 'texmode', 'on')
      | port_label('input', 3, 'V_{A}', 'texmode', 'on')
      | port_label('input', 4, '\omega_{A}', 'texmode', 'on')
      | port_label('input', 5, 'T_{WRA-MAC}', 'texmode', 'on')
      | port_label('input', 6, 'T_{MAC-WRA}', 'texmode', 'on')
      | 
      | port_label('output', 1, 'FM_{A}', 'texmode', 'on')
  Fin Self-Influence : Subsystem
      mask Display:
      | port_label('input', 1, 'Parameters', 'texmode', 'on')
      | port_label('input', 2, 'Environment', 'texmode', 'on')
      | port_label('input', 3, 'V_{A|IERA}', 'texmode', 'on')
      | port_label('input', 4, '\omega_{A|IERA}', 'texmode', 'on')
      | port_label('input', 5, 'FM_{A|IERA}', 'texmode', 'on')
      | 
      | port_label('output', 1, 'd_{k|IERA}', 'texmode', 'on')
  Mux : Mux  Inputs=3
  Sum : Sum  Inputs=|++
  Terminator : Terminator
  Terminator1 : Terminator
  Transpose : Subsystem
      mask Display: disp('A^T', 'texmode', 'on')
  Unary Minus : simulink/Math Operations/Unary Minus  DoSatur=off
  Zero inertial : Constant  Value=[0 0 0 0 0 0]
  FM_I : Outport
  FM_A : Outport  Port=2
  d (k) : Outport  Port=3
  wires:
  Parameters/1 -> Bus Selector/1, Fin/1(Parameters), Fin Self-Influence/1(Parameters)
  Environment/1 -> Fin/2(Environment), Fin Self-Influence/2(Environment)
  Euler Rotation Matrix MAC to WRA (Half Wing)/1 -> Transpose/1(In), Fin/5(T_WRA_MAC)
  Transpose/1(Out) -> Fin/6(T_MAC_WRA)
  Mux/1 -> Euler Rotation Matrix MAC to WRA (Half Wing)/1
  Unary Minus/1 -> Mux/1
  Bus Selector/1 -> Unary Minus/1  "<dihedral>"
  Bus Selector/2 -> Sum/1  "<incid>"
  Bus Selector/3 -> Mux/3  "<sweep>"
  Sum/1 -> Mux/2
  control/1 -> Sum/2
  V_A/1 -> Fin/3(V_A), Fin Self-Influence/3(V_A)
  omega_A/1 -> Fin/4(omega_A), Fin Self-Influence/4(omega_A)
  V_W/1 -> Terminator/1
  omega_W/1 -> Terminator1/1
  Zero inertial/1 -> FM_I/1
  Fin/1(FM_A) -> FM_A/1, Fin Self-Influence/5(FM_A)
  Fin Self-Influence/1(d (k)) -> d (k)/1

== system UAVdesign_net/Subsystem Models/Fin/IELA to CG ==
  R_IELA_B_B : Inport
  FM_IELA : Inport  Port=2
  3x3 Cross Product : UAVdesign_net/Utilities/Math/3x3 Cross Product  SystemSampleTime=-1
  Demux : Demux  Outputs=2
  Mux : Mux  Inputs=2
  Sum : Sum  Inputs=++|
  FM_B : Outport
  wires:
  FM_IELA/1 -> Demux/1
  Mux/1 -> FM_B/1
  Demux/1 -> Mux/1, 3x3 Cross Product/2
  R_IELA_B_B/1 -> 3x3 Cross Product/1
  Demux/2 -> Sum/2
  Sum/1 -> Mux/2
  3x3 Cross Product/1 -> Sum/1

== system UAVdesign_net/Subsystem Models/Fin/IELA to IERA ==
  T_IERA_IELA : Inport
  V_A_IELA : Inport  Port=2
  omega_A_IELA : Inport  Port=3
  V_W_IELA : Inport  Port=4
  omega_W_IELA : Inport  Port=5
  1D : Reshape
  Demux : Demux
  Product : Product  Multiplication=Matrix(*)  RndMeth=Zero
  Vector Concatenate : Concatenate  NumInputs=4  Mode=Multidimensional array  ConcatenateDimension=2
  V_A_IERA : Outport
  omega_A_IERA : Outport  Port=2
  V_W_IERA : Outport  Port=3
  omega_W_IERA : Outport  Port=4
  wires:
  T_IERA_IELA/1 -> Product/1
  V_A_IELA/1 -> Vector Concatenate/1
  omega_A_IELA/1 -> Vector Concatenate/2
  Vector Concatenate/1 -> Product/2
  Product/1 -> 1D/1
  1D/1 -> Demux/1
  Demux/1 -> V_A_IERA/1
  Demux/2 -> omega_A_IERA/1
  Demux/3 -> V_W_IERA/1
  Demux/4 -> omega_W_IERA/1
  V_W_IELA/1 -> Vector Concatenate/3
  omega_W_IELA/1 -> Vector Concatenate/4

== system UAVdesign_net/Subsystem Models/Fin/IERA to IELA ==
  T_IELA_IERA : Inport
  FM_I_IERA : Inport  Port=2
  FM_A_IERA : Inport  Port=3
  d_IERA : Inport  Port=4
  1D : Reshape
  Demux : Demux  Outputs=[6 6 3]
  Demux1 : Demux  Outputs=2
  Demux2 : Demux  Outputs=2
  Product : Product  Multiplication=Matrix(*)  RndMeth=Zero
  Signal Specification{,1..4} (5 alike) : SignalSpecification  Dimensions=3
  Vector Concatenate : Concatenate  NumInputs=5  Mode=Multidimensional array  ConcatenateDimension=2
  FM_I_IELA : Outport
  FM_A_IELA : Outport  Port=2
  d_IELA : Outport  Port=3
  wires:
  T_IELA_IERA/1 -> Product/1
  Vector Concatenate/1 -> Product/2
  Product/1 -> 1D/1
  1D/1 -> Demux/1
  Demux/1 -> FM_I_IELA/1
  Demux/2 -> FM_A_IELA/1
  Demux/3 -> d_IELA/1
  d_IERA/1 -> Signal Specification4/1
  FM_I_IERA/1 -> Demux1/1
  Demux1/2 -> Signal Specification1/1
  Demux1/1 -> Signal Specification/1
  Demux2/1 -> Signal Specification2/1
  Demux2/2 -> Signal Specification3/1
  FM_A_IERA/1 -> Demux2/1
  Signal Specification/1 -> Vector Concatenate/1
  Signal Specification1/1 -> Vector Concatenate/2
  Signal Specification2/1 -> Vector Concatenate/3
  Signal Specification3/1 -> Vector Concatenate/4
  Signal Specification4/1 -> Vector Concatenate/5

== system UAVdesign_net/Subsystem Models/Fin/Transpose ==
  In : Inport
  Permute Dimensions : PermuteDimensions
  Out : Outport
  wires:
  Permute Dimensions/1 -> Out/1
  In/1 -> Permute Dimensions/1

== system UAVdesign_net/Subsystem Models/Fuselage/CG to IELA ==
  R_IELA-B|B : Inport
  V_B-E|B : Inport  Port=2
  omega_B_E|B : Inport  Port=3
  3x3 Cross Product : UAVdesign_net/Utilities/Math/3x3 Cross Product  SystemSampleTime=-1
  Sum : Sum  Inputs=++|
  V_IELA-E|IELA : Outport
  omega_IELA-E|IELA : Outport  Port=2
  wires:
  omega_B_E|B/1 -> 3x3 Cross Product/1, omega_IELA-E|IELA/1
  R_IELA-B|B/1 -> 3x3 Cross Product/2
  3x3 Cross Product/1 -> Sum/2
  V_B-E|B/1 -> Sum/1
  Sum/1 -> V_IELA-E|IELA/1

== system UAVdesign_net/Subsystem Models/Fuselage/Fuselage Model (IERA) ==
  Parameters : Inport  OutDataTypeStr=Bus: FuselageParameters
  Environment : Inport  Port=2  OutDataTypeStr=Bus: Environment
  V_A : Inport  Port=3
  omega_A : Inport  Port=4
  V_W : Inport  Port=5
  omega_W : Inport  Port=6
  Fuselage Forces and Moments : Subsystem
      mask Display:
      | port_label('input', 1, 'Parameters', 'texmode', 'on')
      | port_label('input', 2, 'Environment', 'texmode', 'on')
      | port_label('input', 3, 'V_{A|WRA}', 'texmode', 'on')
      | port_label('input', 4, '\omega_{A|WRA}', 'texmode', 'on')
      | 
      | port_label('output', 1, 'FM_{A}', 'texmode', 'on')
  Fuselage Self-Influence : Subsystem
      mask Display:
      | port_label('input', 1, 'Parameters', 'texmode', 'on')
      | port_label('input', 2, 'Environment', 'texmode', 'on')
      | port_label('input', 3, 'V_{A|IERA}', 'texmode', 'on')
      | port_label('input', 4, '\omega_{A|IERA}', 'texmode', 'on')
      | port_label('input', 5, 'FM_{A|IERA}', 'texmode', 'on')
      | 
      | port_label('output', 1, 'd_{k|IERA}', 'texmode', 'on')
  Terminator : Terminator
  Terminator1 : Terminator
  Zero inertial : Constant  Value=[0 0 0 0 0 0]
  FM_I : Outport
  FM_A : Outport  Port=2
  d (k) : Outport  Port=3
  wires:
  Parameters/1 -> Fuselage Self-Influence/1(Parameters), Fuselage Forces and Moments/1(Parameters)
  Environment/1 -> Fuselage Self-Influence/2(Environment), Fuselage Forces and Moments/2(Environment)
  V_A/1 -> Fuselage Self-Influence/3(V_A), Fuselage Forces and Moments/3(V_A)
  omega_A/1 -> Fuselage Self-Influence/4(omega_A), Fuselage Forces and Moments/4(omega_A)
  V_W/1 -> Terminator/1
  omega_W/1 -> Terminator1/1
  Zero inertial/1 -> FM_I/1
  Fuselage Forces and Moments/1(FM_A) -> FM_A/1, Fuselage Self-Influence/5(FM_A)
  Fuselage Self-Influence/1(d (k)) -> d (k)/1

== system UAVdesign_net/Subsystem Models/Fuselage/IELA to CG ==
  R_IELA_B_B : Inport
  FM_IELA : Inport  Port=2
  3x3 Cross Product : UAVdesign_net/Utilities/Math/3x3 Cross Product  SystemSampleTime=-1
  Demux : Demux  Outputs=2
  Mux : Mux  Inputs=2
  Sum : Sum  Inputs=++|
  FM_B : Outport
  wires:
  FM_IELA/1 -> Demux/1
  Mux/1 -> FM_B/1
  Demux/1 -> Mux/1, 3x3 Cross Product/2
  R_IELA_B_B/1 -> 3x3 Cross Product/1
  Demux/2 -> Sum/2
  Sum/1 -> Mux/2
  3x3 Cross Product/1 -> Sum/1

== system UAVdesign_net/Subsystem Models/Fuselage/IELA to IERA ==
  T_IERA_IELA : Inport
  V_A_IELA : Inport  Port=2
  omega_A_IELA : Inport  Port=3
  V_W_IELA : Inport  Port=4
  omega_W_IELA : Inport  Port=5
  1D : Reshape
  Demux : Demux
  Product : Product  Multiplication=Matrix(*)  RndMeth=Zero
  Vector Concatenate : Concatenate  NumInputs=4  Mode=Multidimensional array  ConcatenateDimension=2
  V_A_IERA : Outport
  omega_A_IERA : Outport  Port=2
  V_W_IERA : Outport  Port=3
  omega_W_IERA : Outport  Port=4
  wires:
  T_IERA_IELA/1 -> Product/1
  V_A_IELA/1 -> Vector Concatenate/1
  omega_A_IELA/1 -> Vector Concatenate/2
  Vector Concatenate/1 -> Product/2
  Product/1 -> 1D/1
  1D/1 -> Demux/1
  Demux/1 -> V_A_IERA/1
  Demux/2 -> omega_A_IERA/1
  Demux/3 -> V_W_IERA/1
  Demux/4 -> omega_W_IERA/1
  V_W_IELA/1 -> Vector Concatenate/3
  omega_W_IELA/1 -> Vector Concatenate/4

== system UAVdesign_net/Subsystem Models/Fuselage/IERA to IELA ==
  T_IELA_IERA : Inport
  FM_I_IERA : Inport  Port=2
  FM_A_IERA : Inport  Port=3
  d_IERA : Inport  Port=4
  1D : Reshape
  Demux : Demux  Outputs=[6 6 3]
  Demux1 : Demux  Outputs=2
  Demux2 : Demux  Outputs=2
  Product : Product  Multiplication=Matrix(*)  RndMeth=Zero
  Signal Specification{,1..4} (5 alike) : SignalSpecification  Dimensions=3
  Vector Concatenate : Concatenate  NumInputs=5  Mode=Multidimensional array  ConcatenateDimension=2
  FM_I_IELA : Outport
  FM_A_IELA : Outport  Port=2
  d_IELA : Outport  Port=3
  wires:
  T_IELA_IERA/1 -> Product/1
  Vector Concatenate/1 -> Product/2
  Product/1 -> 1D/1
  1D/1 -> Demux/1
  Demux/1 -> FM_I_IELA/1
  Demux/2 -> FM_A_IELA/1
  Demux/3 -> d_IELA/1
  d_IERA/1 -> Signal Specification4/1
  FM_I_IERA/1 -> Demux1/1
  Demux1/2 -> Signal Specification1/1
  Demux1/1 -> Signal Specification/1
  Demux2/1 -> Signal Specification2/1
  Demux2/2 -> Signal Specification3/1
  FM_A_IERA/1 -> Demux2/1
  Signal Specification/1 -> Vector Concatenate/1
  Signal Specification1/1 -> Vector Concatenate/2
  Signal Specification2/1 -> Vector Concatenate/3
  Signal Specification3/1 -> Vector Concatenate/4
  Signal Specification4/1 -> Vector Concatenate/5

== system UAVdesign_net/Subsystem Models/Fuselage/Transpose ==
  In : Inport
  Permute Dimensions : PermuteDimensions
  Out : Outport
  wires:
  Permute Dimensions/1 -> Out/1
  In/1 -> Permute Dimensions/1

== system UAVdesign_net/Subsystem Models/Helicopter Parameters/Fin Parameters ==
  In : Inport
  Bus Creator : BusCreator  Inputs=14  OutDataTypeStr=Bus: FinParameters  NonVirtualBus=on
  Demux : Demux  Outputs=14
  Gain{,1..3} (4 alike) : Gain  Gain=pi/180
  Parameters : Outport  OutDataTypeStr=Bus: FinParameters
  wires:
  Demux/14 -> Bus Creator/14  "cm1s1"
  Demux/13 -> Bus Creator/13  "cm0"
  Demux/12 -> Bus Creator/12  "cd2c1"
  Demux/11 -> Bus Creator/11  "cd1s1"
  Demux/10 -> Bus Creator/10  "cd0"
  Demux/9 -> Bus Creator/9  "a1s2"
  Demux/8 -> Bus Creator/8  "a0"
  Gain3/1 -> Bus Creator/7  "stall"
  Demux/7 -> Gain3/1
  Demux/6 -> Bus Creator/6  "taper"
  Demux/5 -> Gain1/1
  Gain1/1 -> Bus Creator/5  "sweep"
  Gain/1 -> Bus Creator/4  "incid"
  Demux/4 -> Gain/1
  Gain2/1 -> Bus Creator/3  "dihedral"
  Demux/3 -> Gain2/1
  Demux/2 -> Bus Creator/2  "chord"
  Demux/1 -> Bus Creator/1  "span"
  Bus Creator/1 -> Parameters/1
  In/1 -> Demux/1

== system UAVdesign_net/Subsystem Models/Helicopter Parameters/Fin Parameters1 ==
  In : Inport
  Bus Creator : BusCreator  Inputs=14  OutDataTypeStr=Bus: FinParameters  NonVirtualBus=on
  Demux : Demux  Outputs=14
  Gain{,1..3} (4 alike) : Gain  Gain=pi/180
  Parameters : Outport  OutDataTypeStr=Bus: FinParameters
  wires:
  In/1 -> Demux/1
  Bus Creator/1 -> Parameters/1
  Demux/1 -> Bus Creator/1  "span"
  Demux/2 -> Bus Creator/2  "chord"
  Demux/3 -> Gain2/1
  Gain2/1 -> Bus Creator/3  "dihedral"
  Demux/4 -> Gain/1
  Gain/1 -> Bus Creator/4  "incid"
  Gain1/1 -> Bus Creator/5  "sweep"
  Demux/5 -> Gain1/1
  Demux/6 -> Bus Creator/6  "taper"
  Demux/7 -> Gain3/1
  Gain3/1 -> Bus Creator/7  "stall"
  Demux/8 -> Bus Creator/8  "a0"
  Demux/9 -> Bus Creator/9  "a1s2"
  Demux/10 -> Bus Creator/10  "cd0"
  Demux/11 -> Bus Creator/11  "cd1s1"
  Demux/12 -> Bus Creator/12  "cd2c1"
  Demux/13 -> Bus Creator/13  "cm0"
  Demux/14 -> Bus Creator/14  "cm1s1"

== system UAVdesign_net/Subsystem Models/Helicopter Parameters/Fuse Parameters ==
  In : Inport
  Bus Creator : BusCreator  Inputs=7  OutDataTypeStr=Bus: FuselageParameters  NonVirtualBus=on
  Demux : Demux  Outputs=17
  Vector Concatenate{,1..4} (5 alike) : Concatenate  NumInputs=3  Mode=Vector
  Parameters : Outport  OutDataTypeStr=Bus: FuselageParameters
  wires:
  Vector Concatenate4/1 -> Bus Creator/7  "cn"
  Vector Concatenate3/1 -> Bus Creator/6  "cm"
  Demux/17 -> Vector Concatenate4/3
  Demux/16 -> Vector Concatenate4/2
  Demux/15 -> Vector Concatenate4/1
  Demux/14 -> Vector Concatenate3/3
  Demux/13 -> Vector Concatenate3/2
  Demux/12 -> Vector Concatenate3/1
  Vector Concatenate2/1 -> Bus Creator/5  "cz"
  Demux/11 -> Vector Concatenate2/3
  Demux/10 -> Vector Concatenate2/2
  Demux/9 -> Vector Concatenate2/1
  Vector Concatenate1/1 -> Bus Creator/4  "cy"
  Demux/8 -> Vector Concatenate1/3
  Demux/7 -> Vector Concatenate1/2
  Demux/6 -> Vector Concatenate1/1
  Vector Concatenate/1 -> Bus Creator/3  "cx"
  Demux/5 -> Vector Concatenate/3
  Demux/4 -> Vector Concatenate/2
  Demux/3 -> Vector Concatenate/1
  Demux/2 -> Bus Creator/2  "clen"
  In/1 -> Demux/1
  Bus Creator/1 -> Parameters/1
  Demux/1 -> Bus Creator/1  "carea"

== system UAVdesign_net/Subsystem Models/Helicopter Parameters/Rotor Parameters ==
  In : Inport
  Bus Creator : BusCreator  Inputs=18  OutDataTypeStr=Bus: RotorParameters  NonVirtualBus=on
  Data Type Conversion : DataTypeConversion  OutDataTypeStr=int32  RndMeth=Nearest
  Data Type Conversion1 : DataTypeConversion  OutDataTypeStr=uint32  RndMeth=Nearest
  Demux : Demux  Outputs=20
  Gain : Gain  Gain=pi/180
  Gain1 : Gain  Gain=pi/180
  Gain2 : Gain  Gain=180/pi
  Gain3 : Gain  Gain=pi/180
  Vector Concatenate : Concatenate  NumInputs=3  Mode=Vector
  Parameters : Outport  OutDataTypeStr=Bus: RotorParameters
  wires:
  Demux/14 -> Bus Creator/12  "btq"
  Demux/15 -> Gain3/1
  Demux/12 -> Bus Creator/10  "btmin"
  Demux/11 -> Bus Creator/9  "chord"
  Demux/10 -> Bus Creator/8  "radius"
  Demux/9 -> Data Type Conversion1/1
  Data Type Conversion1/1 -> Bus Creator/7  "nb"
  Demux/8 -> Gain2/1
  Demux/7 -> Bus Creator/5  "e"
  Demux/6 -> Gain1/1
  Demux/5 -> Gain/1
  Gain3/1 -> Bus Creator/13  "twist"
  Gain2/1 -> Bus Creator/6  "khub"
  Gain1/1 -> Bus Creator/4  "delta3"
  Gain/1 -> Bus Creator/3  "precone"
  Demux/19 -> Data Type Conversion/1
  Data Type Conversion/1 -> Bus Creator/17  "hubtype"
  In/1 -> Demux/1
  Vector Concatenate/1 -> Bus Creator/2  "del0_2"
  Demux/2 -> Vector Concatenate/1
  Demux/3 -> Vector Concatenate/2
  Demux/4 -> Vector Concatenate/3
  Bus Creator/1 -> Parameters/1
  Demux/1 -> Bus Creator/1  "a0"
  Demux/13 -> Bus Creator/11  "btmax"
  Demux/16 -> Bus Creator/14  "iflap"
  Demux/17 -> Bus Creator/15  "mbar"
  Demux/18 -> Bus Creator/16  "lmast"
  Demux/20 -> Bus Creator/18  "azsign"

== system UAVdesign_net/Subsystem Models/Helicopter Parameters/Rotor Parameters1 ==
  In : Inport
  Bus Creator : BusCreator  Inputs=18  OutDataTypeStr=Bus: RotorParameters  NonVirtualBus=on
  Data Type Conversion : DataTypeConversion  OutDataTypeStr=int32  RndMeth=Nearest
  Data Type Conversion1 : DataTypeConversion  OutDataTypeStr=uint32  RndMeth=Nearest
  Demux : Demux  Outputs=20
  Gain : Gain  Gain=pi/180
  Gain1 : Gain  Gain=pi/180
  Gain2 : Gain  Gain=180/pi
  Gain3 : Gain  Gain=pi/180
  Vector Concatenate : Concatenate  NumInputs=3  Mode=Vector
  Parameters : Outport  OutDataTypeStr=Bus: RotorParameters
  wires:
  Demux/20 -> Bus Creator/18  "azsign"
  Demux/18 -> Bus Creator/16  "lmast"
  Demux/17 -> Bus Creator/15  "mbar"
  Demux/16 -> Bus Creator/14  "iflap"
  Demux/13 -> Bus Creator/11  "btmax"
  Demux/1 -> Bus Creator/1  "a0"
  Bus Creator/1 -> Parameters/1
  Demux/4 -> Vector Concatenate/3
  Demux/3 -> Vector Concatenate/2
  Demux/2 -> Vector Concatenate/1
  Vector Concatenate/1 -> Bus Creator/2  "del0_2"
  In/1 -> Demux/1
  Data Type Conversion/1 -> Bus Creator/17  "hubtype"
  Demux/19 -> Data Type Conversion/1
  Gain/1 -> Bus Creator/3  "precone"
  Gain1/1 -> Bus Creator/4  "delta3"
  Gain2/1 -> Bus Creator/6  "khub"
  Gain3/1 -> Bus Creator/13  "twist"
  Demux/5 -> Gain/1
  Demux/6 -> Gain1/1
  Demux/7 -> Bus Creator/5  "e"
  Demux/8 -> Gain2/1
  Data Type Conversion1/1 -> Bus Creator/7  "nb"
  Demux/9 -> Data Type Conversion1/1
  Demux/10 -> Bus Creator/8  "radius"
  Demux/11 -> Bus Creator/9  "chord"
  Demux/12 -> Bus Creator/10  "btmin"
  Demux/15 -> Gain3/1
  Demux/14 -> Bus Creator/12  "btq"

== system UAVdesign_net/Subsystem Models/Helicopter Rotor/CG to IELA ==
  R_IELA-B|B : Inport
  V_B-E|B : Inport  Port=2
  omega_B_E|B : Inport  Port=3
  V_dot_B-E|B : Inport  Port=4
  omega_dot_B-E|B : Inport  Port=5
  3x3 Cross Product : UAVdesign_net/Utilities/Math/3x3 Cross Product  SystemSampleTime=-1
  3x3 Cross Product1 : UAVdesign_net/Utilities/Math/3x3 Cross Product  SystemSampleTime=-1
  Sum : Sum  Inputs=++|
  Sum1 : Sum  Inputs=|++
  V_IELA-E|IELA : Outport
  omega_IELA-E|IELA : Outport  Port=2
  V_dot_IELA-E|IELA : Outport  Port=3
  omega_dot_IELA-E|IELA : Outport  Port=4
  wires:
  Sum1/1 -> V_dot_IELA-E|IELA/1
  V_dot_B-E|B/1 -> Sum1/2
  3x3 Cross Product1/1 -> Sum1/1
  omega_dot_B-E|B/1 -> omega_dot_IELA-E|IELA/1, 3x3 Cross Product1/1
  Sum/1 -> V_IELA-E|IELA/1
  V_B-E|B/1 -> Sum/1
  3x3 Cross Product/1 -> Sum/2
  R_IELA-B|B/1 -> 3x3 Cross Product1/2, 3x3 Cross Product/2
  omega_B_E|B/1 -> omega_IELA-E|IELA/1, 3x3 Cross Product/1

== system UAVdesign_net/Subsystem Models/Helicopter Rotor/Direction of Rotation ==
  Parameters : Inport  OutDataTypeStr=Bus: RotorParameters
  V_B-E|B_in : Inport  Port=2
  omega_B_E|B_in : Inport  Port=3
  V_dot_B-E|B_in : Inport  Port=4
  omega_dot_B-E|B_in : Inport  Port=5
  Bus Selector : BusSelector  OutputSignals=azsign
  Constant : Constant
  Mux : Mux  Inputs=3
  Mux1 : Mux  Inputs=3
  Product{,1..3} (4 alike) : Product  RndMeth=Zero
  Unary Minus : simulink/Math Operations/Unary Minus  DoSatur=off
  V_B-E|B : Outport
  omega_B_E|B : Outport  Port=2
  V_dot_B-E|B : Outport  Port=3
  omega_dot_B-E|B : Outport  Port=4
  wires:
  Product2/1 -> omega_B_E|B/1
  Product3/1 -> omega_dot_B-E|B/1
  omega_dot_B-E|B_in/1 -> Product3/2
  omega_B_E|B_in/1 -> Product2/2
  Mux/1 -> Product3/1, Product2/1
  Product1/1 -> V_dot_B-E|B/1
  V_dot_B-E|B_in/1 -> Product1/2
  Mux1/1 -> Product1/1, Product/1
  Product/1 -> V_B-E|B/1
  V_B-E|B_in/1 -> Product/2
  Constant/1 -> Mux1/3, Mux1/1, Mux/2
  Unary Minus/1 -> Mux1/2, Mux/3, Mux/1
  Bus Selector/1 -> Unary Minus/1  "<azsign>"
  Parameters/1 -> Bus Selector/1

== system UAVdesign_net/Subsystem Models/Helicopter Rotor/Direction of Rotation 2 ==
  Parameters : Inport  OutDataTypeStr=Bus: RotorParameters
  FM_A_IERA_in : Inport  Port=2
  d_IERA_in : Inport  Port=3
  Bus Selector : BusSelector  OutputSignals=azsign
  Constant : Constant
  Mux : Mux  Inputs=6
  Mux1 : Mux  Inputs=3
  Product : Product  RndMeth=Zero
  Product1 : Product  RndMeth=Zero
  Unary Minus : simulink/Math Operations/Unary Minus  DoSatur=off
  FM_A_IERA : Outport
  d_IERA : Outport  Port=2
  wires:
  d_IERA_in/1 -> Product1/2
  Product1/1 -> d_IERA/1
  Mux1/1 -> Product1/1
  Mux/1 -> Product/1
  Constant/1 -> Mux1/3, Mux1/1, Mux/5, Mux/3, Mux/1
  Unary Minus/1 -> Mux1/2, Mux/6, Mux/4, Mux/2
  Parameters/1 -> Bus Selector/1
  Bus Selector/1 -> Unary Minus/1  "<azsign>"
  FM_A_IERA_in/1 -> Product/2
  Product/1 -> FM_A_IERA/1

== system UAVdesign_net/Subsystem Models/Helicopter Rotor/IELA to CG ==
  R_IELA_B_B : Inport
  FM_IELA : Inport  Port=2
  3x3 Cross Product : UAVdesign_net/Utilities/Math/3x3 Cross Product  SystemSampleTime=-1
  Demux : Demux  Outputs=2
  Mux : Mux  Inputs=2
  Sum : Sum  Inputs=++|
  FM_B : Outport
  wires:
  3x3 Cross Product/1 -> Sum/1
  Sum/1 -> Mux/2
  Demux/2 -> Sum/2
  R_IELA_B_B/1 -> 3x3 Cross Product/1
  Demux/1 -> 3x3 Cross Product/2, Mux/1
  Mux/1 -> FM_B/1
  FM_IELA/1 -> Demux/1

== system UAVdesign_net/Subsystem Models/Helicopter Rotor/IELA to IERA ==
  T_IERA_IELA : Inport
  V_I_IELA : Inport  Port=2
  omega_I_IELA : Inport  Port=3
  V_dot_I_IELA : Inport  Port=4
  omega_dot_I_IELA : Inport  Port=5
  V_A_IELA : Inport  Port=6
  omega_A_IELA : Inport  Port=7
  1D : Reshape
  Demux : Demux  Outputs=6
  Product : Product  Multiplication=Matrix(*)  RndMeth=Zero
  Vector Concatenate : Concatenate  NumInputs=6  Mode=Multidimensional array  ConcatenateDimension=2
  V_I_IERA : Outport
  omega_I_IERA : Outport  Port=2
  V_dot_I_IERA : Outport  Port=3
  omega_dot_I_IERA : Outport  Port=4
  V_A_IERA : Outport  Port=5
  omega_A_IERA : Outport  Port=6
  wires:
  Demux/6 -> omega_A_IERA/1
  Demux/5 -> V_A_IERA/1
  Demux/4 -> omega_dot_I_IERA/1
  Demux/3 -> V_dot_I_IERA/1
  Demux/2 -> omega_I_IERA/1
  Demux/1 -> V_I_IERA/1
  1D/1 -> Demux/1
  Product/1 -> 1D/1
  Vector Concatenate/1 -> Product/2
  omega_A_IELA/1 -> Vector Concatenate/6
  V_A_IELA/1 -> Vector Concatenate/5
  omega_dot_I_IELA/1 -> Vector Concatenate/4
  V_dot_I_IELA/1 -> Vector Concatenate/3
  omega_I_IELA/1 -> Vector Concatenate/2
  V_I_IELA/1 -> Vector Concatenate/1
  T_IERA_IELA/1 -> Product/1
